simulink model "SimulinkAnalysisofCheetahTail"  (R2022a)
settings: Solver=ode4  StartTime=0.0  StopTime=1.5  FixedStep=0.001  RelTol=1e-3
undefined symbols (not defined in the file): B_cg_H, B_con_H, B_con_L, bar_len, cd_table, Cf, cl_table, g, gear_ratio, int_point_bar, int_point_tail, ITail, M_add, M_cg_H, M_cg_L, M_cg_W, Mb, Mm, Mt, psi3, rho, T_cg_H, T_fur_gap, T_length, T_width_major, T_width_minor, th2_initial, torque_constant, uncertainty_Forces, uncertainty_Position, Vf, windspeed
(part 11 of 21)

== matlab function SimulinkAnalysisofCheetahTail/Model/GravityMatrix ==
  data: B_cg_H parameter; B_con_H parameter; B_con_L parameter; M_cg_H parameter; M_cg_L parameter; M_cg_W parameter; Mb parameter; Mm parameter; Mt parameter; T_cg_H parameter; g parameter; G output; q input
function G = GravityMatrix(B_cg_H,B_con_H,B_con_L,M_cg_H,M_cg_L,M_cg_W,Mb,Mm,Mt,T_cg_H,g,q)
%#codegen
[x,y,z,phi1,th1,psi1,phi2,th2] = deal(q(1),q(2),q(3),q(4),q(5),q(6),q(7),q(8));
% [dx,dy,dz,dphi1,dth1,dpsi1,dphi2,dth2] = deal(dq(1),dq(2),dq(3),dq(4),dq(5),dq(6),dq(7),dq(8));
%    This function was generated by the Symbolic Math Toolbox version 9.0.
%    26-Jan-2022 10:48:01

t2 = cos(phi1);
t3 = cos(phi2);
t4 = cos(th1);
t5 = cos(th2);
t6 = sin(phi1);
t7 = sin(phi2);
t8 = sin(th1);
t9 = sin(th2);
t10 = M_cg_L+x;
t11 = M_cg_W+y;
t12 = M_cg_H+z;
t13 = B_con_L.*t4;
t14 = t4.*t10;
t15 = B_con_H.*t2.*t8;
t16 = B_con_H.*t4.*t6;
t17 = t6.*t7.*t8;
t18 = t7.*t8.*t9;
t19 = t2.*t4.*t7;
t20 = t3.*t4.*t6;
t21 = t3.*t4.*t9;
t22 = t3.*t5.*t8;
t23 = t2.*t4.*t11;
t24 = t2.*t8.*t12;
t25 = t4.*t6.*t12;
t26 = t6.*t8.*t11;
t27 = -t15;
t28 = -t17;
t29 = -t18;
t30 = t2.*t21;
t31 = t2.*t22;
t32 = t5.*t19;
t33 = t5.*t20;
t34 = -t24;
t35 = t19+t33;
t36 = t22+t30;
t37 = t21+t28+t31;
t38 = t20+t29+t32;
mt1 = [Mb.*g.*t8+Mm.*g.*t8+Mt.*g.*t8;-Mb.*g.*t4.*t6-Mm.*g.*t4.*t6-Mt.*g.*t4.*t6;Mb.*g.*t2.*t4+Mm.*g.*t2.*t4+Mt.*g.*t2.*t4;-Mm.*g.*(t23+t25)-Mt.*g.*(t16-t19.*(2.7e+1./1.0e+2)+t23+t25-t33.*(2.7e+1./1.0e+2)-T_cg_H.*t35)-Mb.*g.*(t16+t23+t25-B_cg_H.*t35);Mt.*g.*(t13+t14-t17.*(2.7e+1./1.0e+2)+t21.*(2.7e+1./1.0e+2)+t26+t27+t31.*(2.7e+1./1.0e+2)+t34+T_cg_H.*t37)+Mb.*g.*(t13+t14+t26+t27+t34+B_cg_H.*t37)+Mm.*g.*(t14+t26+t34);0.0];
mt2 = [Mt.*g.*(t18.*(-2.7e+1./1.0e+2)+t20.*(2.7e+1./1.0e+2)+t32.*(2.7e+1./1.0e+2)+T_cg_H.*t38)+B_cg_H.*Mb.*g.*t38;Mt.*g.*(t22.*(2.7e+1./1.0e+2)+t30.*(2.7e+1./1.0e+2)+T_cg_H.*t36)+B_cg_H.*Mb.*g.*t36];
G = [mt1;mt2];

== matlab function SimulinkAnalysisofCheetahTail/Model/ConstraintJacobian ==
  data: A output
function A = ConstraintJacobian
%#codegen

%    This function was generated by the Symbolic Math Toolbox version 9.0.
%    26-Jan-2022 10:48:03

A = reshape([1.0,0.0,0.0,0.0,0.0,0.0,0.0,0.0,1.0,0.0,0.0,0.0,0.0,0.0,0.0,0.0,1.0,0.0,0.0,0.0,0.0,0.0,0.0,0.0,1.0,0.0,0.0,0.0,0.0,0.0,0.0,0.0,1.0,0.0,0.0,0.0,0.0,0.0,0.0,0.0,1.0,0.0,0.0,0.0,0.0,0.0,0.0,0.0,0.0,0.0,0.0,0.0,0.0,0.0,0.0,1.0],[7,8]);

== matlab function SimulinkAnalysisofCheetahTail/Model/ConstraintJacobianDeriv ==
  data: dA output
function dA = ConstraintJacobianDeriv
%#codegen

%    This function was generated by the Symbolic Math Toolbox version 9.0.
%    26-Jan-2022 10:48:04

dA = reshape([0.0,0.0,0.0,0.0,0.0,0.0,0.0,0.0,0.0,0.0,0.0,0.0,0.0,0.0,0.0,0.0,0.0,0.0,0.0,0.0,0.0,0.0,0.0,0.0,0.0,0.0,0.0,0.0,0.0,0.0,0.0,0.0,0.0,0.0,0.0,0.0,0.0,0.0,0.0,0.0,0.0,0.0,0.0,0.0,0.0,0.0,0.0,0.0,0.0,0.0,0.0,0.0,0.0,0.0,0.0,0.0],[7,8]);

== matlab function SimulinkAnalysisofCheetahTail/Model/CalculateLambda ==
  data: M input; lambda output; C input; G input; A input; dA input; Q input; tor input; dq input
function lambda= calcLambda(M,C,G,A,dA,Q, tor, dq)

B = [0;0;0;0;0;0;1;0];
% lambda = -(A*inv(M)*A')\(A*inv(M)*(-C*dq-G)+ dA*dq);
lambda = -((A/M)*A')\((A/M)*(B*tor-C-G-Q)+ dA*dq);

== matlab function SimulinkAnalysisofCheetahTail/Model/Dynamics ==
  data: M input; ddq output; C input; G input; A input; Q input; tor input; lambda input
function ddq = dynamics(M,C,G,A,Q, tor, lambda)
B = [0;0;0;0;0;0;1;0];
% ddq = M\(A'*lambda-C*dq-G);
ddq = M\(A'*lambda+B*tor-C-G-Q);

== matlab function SimulinkAnalysisofCheetahTail/Model/Forces/MATLAB Function ==
  data: int_point_bar input; A_output output; bar_len parameter
function A_output = fcn(int_point_bar, bar_len)

A_output = (bar_len-int_point_bar)*0.02;

== matlab function SimulinkAnalysisofCheetahTail/Model/Forces/NonConstraintForceMatrix_fr ==
  data: Cf parameter; Vf parameter; Q_fr output; q input; dq input
function Q_fr = NonConstraintForceMatrix_fr(Cf,Vf,q, dq)
%#codegen
[x,y,z,phi1,th1,psi1,phi2,th2] = deal(q(1),q(2),q(3),q(4),q(5),q(6),q(7),q(8));
[dx,dy,dz,dphi1,dth1,dpsi1,dphi2,dth2] = deal(dq(1),dq(2),dq(3),dq(4),dq(5),dq(6),dq(7),dq(8));
%    This function was generated by the Symbolic Math Toolbox version 9.0.
%    10-Feb-2022 10:56:36

t2 = cos(psi1);
t3 = cos(th1);
t4 = sin(psi1);
t5 = sin(th1);
t6 = Vf.*dphi2;
t10 = dphi2.*1.0e+1;
t7 = t2.^2;
t8 = t3.^2;
t9 = t4.^2;
t11 = tanh(t10);
t12 = Cf.*t11;
t13 = t6+t12;
Q_fr = [0.0;0.0;0.0;0.0;phi2.*t3.*t5.*t13-phi2.*t3.*t5.*t7.*t13-phi2.*t3.*t5.*t9.*t13;0.0;t5.^2.*t13+t7.*t8.*t13+t8.*t9.*t13;0.0];

== matlab function SimulinkAnalysisofCheetahTail/Model/Forces/NonConstraintForceMatrix_bar ==
  data: B_con_H parameter; B_con_L parameter; M_cg_H parameter; M_cg_L parameter; M_cg_W parameter; area_bar_drag input; bar_len parameter; int_point_bar input; psi3 parameter; rho parameter; windspeed parameter; q input; dq input; Q_bar output
function Q_bar = NonConstraintForceMatrix_bar(B_con_H,B_con_L,M_cg_H,M_cg_L,M_cg_W,area_bar_drag,bar_len,int_point_bar,psi3,rho,windspeed,q,dq)
%#codegen
[x,y,z,phi1,th1,psi1,phi2,th2] = deal(q(1),q(2),q(3),q(4),q(5),q(6),q(7),q(8));
[dx,dy,dz,dphi1,dth1,dpsi1,dphi2,dth2] = deal(dq(1),dq(2),dq(3),dq(4),dq(5),dq(6),dq(7),dq(8));
%    This function was generated by the Symbolic Math Toolbox version 9.0.
%    09-Feb-2022 08:48:45

t2 = cos(phi1);
t3 = cos(phi2);
t4 = cos(psi1);
t5 = cos(psi3);
t6 = cos(th1);
t7 = cos(th2);
t8 = sin(phi1);
t9 = sin(phi2);
t10 = sin(psi1);
t11 = sin(psi3);
t12 = sin(th1);
t13 = sin(th2);
t14 = M_cg_L+x;
t15 = M_cg_W+y;
t16 = M_cg_H+z;
t26 = bar_len./2.0;
t27 = int_point_bar./2.0;
t17 = B_con_L.*t6;
t18 = B_con_L.*t12;
t19 = t2.*t4;
t20 = t6.*t7;
t21 = t2.*t10;
t22 = t4.*t8;
t23 = t7.*t12;
t24 = t8.*t10;
t25 = t12.*t13;
t28 = B_con_H.*t2.*t6;
t30 = t6.*t14;
t31 = B_con_H.*t2.*t12;
t32 = B_con_H.*t6.*t8;
t35 = t12.*t14;
t39 = t6.*t9.*t13;
t41 = t6.*t10.*t13;
t43 = t8.*t9.*t12;
t46 = t2.*t3.*t6;
t49 = t2.*t6.*t9;
t50 = t3.*t6.*t8;
t52 = t2.*t6.*t13;
t53 = t3.*t6.*t13;
t55 = t4.*t6.*t13;
t58 = t3.*t8.*t12;
t59 = t6.*t8.*t9;
t64 = t2.*t6.*t15;
t66 = t2.*t6.*t16;
t69 = t6.*t8.*t15;
t70 = t2.*t12.*t16;
t71 = t6.*t8.*t16;
t73 = t8.*t12.*t15;
t127 = t26+t27;
t29 = t4.*t17;
t33 = t4.*t18;
t34 = t10.*t17;
t36 = t10.*t18;
t37 = t2.*t25;
t38 = t3.*t25;
t40 = t9.*t23;
t42 = t10.*t23;
t44 = t12.*t24;
t45 = t9.*t25;
t47 = t2.*t20;
t48 = t4.*t20;
t51 = t12.*t19;
t54 = t3.*t23;
t56 = t4.*t23;
t57 = t10.*t20;
t60 = t12.*t21;
t61 = t12.*t22;
t62 = B_con_H.*t6.*t19;
t63 = t4.*t30;
t65 = B_con_H.*t6.*t21;
t67 = t4.*t35;
t68 = t10.*t30;
t72 = t10.*t35;
t74 = -t31;
t77 = -t43;
t82 = t3.*t6.*t22;
t83 = t13.*t46;
t86 = t3.*t8.*t20;
t87 = t6.*t13.*t19;
t88 = t4.*t53;
t91 = t3.*t6.*t24;
t92 = t6.*t9.*t22;
t93 = t2.*t39;
t95 = t8.*t9.*t20;
t96 = t6.*t13.*t21;
t98 = t3.*t41;
t99 = t4.*t39;
t101 = t6.*t9.*t24;
t105 = t10.*t39;
t107 = -t55;
t110 = t6.*t16.*t19;
t111 = t6.*t15.*t22;
t112 = t6.*t16.*t21;
t113 = t6.*t15.*t24;
t115 = -t69;
t116 = -t70;
t117 = t3.*t19.*t20;
t118 = t3.*t20.*t21;
t119 = t9.*t19.*t20;
t120 = t9.*t20.*t21;
t131 = t23+t52;
t75 = -t34;
t76 = -t37;
t78 = -t44;
t79 = -t45;
t80 = t3.*t47;
t81 = t3.*t48;
t84 = t2.*t54;
t85 = t9.*t47;
t89 = t3.*t57;
t90 = t9.*t48;
t94 = t2.*t40;
t97 = t4.*t38;
t100 = t9.*t57;
t102 = -t47;
t103 = t10.*t38;
t104 = t4.*t45;
t106 = -t51;
t108 = -t57;
t109 = t10.*t45;
t114 = -t68;
t122 = -t88;
t124 = -t95;
t129 = -t111;
t130 = -t113;
t132 = t21+t61;
t133 = t22+t60;
t134 = -t117;
t135 = -t118;
t145 = t12.*t131;
t149 = t49+t86;
t152 = t54+t83;
t153 = t56+t87;
t154 = t40+t93;
t155 = t42+t96;
t160 = t2.*t6.*t131;
t163 = t6.*t8.*t131;
t121 = -t80;
t123 = -t89;
t125 = -t100;
t126 = t4.*t79;
t128 = t10.*t79;
t136 = B_con_H.*t132;
t137 = B_con_H.*t133;
t138 = t20+t76;
t139 = t25+t102;
t140 = t19+t78;
t141 = t24+t106;
t142 = t3.*t132;
t143 = t3.*t133;
t144 = t7.*t133;
t146 = t9.*t132;
t147 = t9.*t133;
t148 = t13.*t133;
t156 = t15.*t132;
t157 = t15.*t133;
t158 = t16.*t132;
t159 = t16.*t133;
t174 = t46+t124;
t183 = -t163;
t193 = t39+t58+t94;
t196 = t53+t77+t84;
t197 = t50+t79+t85;
t201 = t127.*t149;
t218 = t92+t97+t134;
t221 = t101+t103+t135;
t234 = t127.*t131.*t152;
t150 = B_con_H.*t140;
t151 = B_con_H.*t141;
t161 = t7.*t142;
t162 = t7.*t143;
t164 = t13.*t143;
t165 = t7.*t146;
t166 = t9.*t144;
t167 = t13.*t147;
t168 = t3.*t140;
t169 = t3.*t141;
t170 = t7.*t141;
t171 = t9.*t140;
t172 = t9.*t141;
t173 = t13.*t141;
t175 = t15.*t140;
t176 = t15.*t141;
t177 = -t157;
t178 = t16.*t140;
t179 = t16.*t141;
t192 = t41+t144;
t194 = t108+t148;
t195 = t38+t59+t121;
t199 = t197.^2;
t203 = t12.*t197;
t206 = -t5.*windspeed.*(t57-t148);
t212 = -t6.*t10.*(t57-t148);
t213 = t2.*t6.*t197;
t215 = t6.*t8.*t197;
t216 = -t201;
t219 = t82+t119+t126;
t222 = t91+t120+t128;
t224 = t6.*t10.*(t57-t148);
t228 = t127.*t196;
t233 = -t133.*(t57-t148);
t236 = -t140.*(t57-t148);
t237 = t127.*t221;
t238 = t127.*t218;
t249 = t127.*t131.*t197;
t260 = t127.*t152.*t197;
t180 = t7.*t168;
t181 = t7.*t169;
t182 = -t161;
t184 = t13.*t169;
t185 = t7.*t171;
t186 = t9.*t170;
t187 = t13.*t172;
t188 = -t168;
t189 = -t176;
t198 = t48+t173;
t200 = t107+t170;
t202 = t12.*t195;
t205 = t123+t164;
t209 = t125+t167;
t211 = t2.*t6.*t195;
t214 = t6.*t8.*t195;
t217 = -t203;
t226 = t165+t169;
t227 = t127.*t195;
t231 = t127.*t199;
t239 = t98+t162+t171;
t248 = -t127.*(t161-t172);
t257 = t32+t64+t71+t216;
t261 = -t260;
t279 = t127.*(t57-t148).*(t89-t164);
t284 = t17+t30+t73+t74+t116+t228;
t296 = t33+t62+t67+t110+t129+t238;
t300 = t36+t65+t72+t112+t130+t237;
t190 = -t180;
t191 = -t186;
t204 = t81+t184;
t207 = t11.*t198.*windspeed;
t208 = t90+t187;
t210 = t4.*t6.*t198;
t223 = -t211;
t225 = t143+t185;
t230 = t172+t182;
t232 = t132.*t198;
t235 = t141.*t198;
t240 = t122+t146+t181;
t242 = t105+t166+t188;
t243 = t5.*t239.*windspeed;
t246 = t6.*t10.*t239;
t259 = t152.*t227;
t262 = t127.*t239;
t263 = t133.*t239;
t270 = t140.*t239;
t276 = t197.*t227;
t280 = t131.*t257;
t283 = t18+t28+t35+t66+t115+t227;
t286 = t195.*t257;
t287 = t197.*t257;
t299 = t131.*t284;
t319 = t195.*t284;
t320 = t197.*t284;
t324 = t136+t158+t189+t248;
t330 = -t300.*(t57-t148);
t331 = t198.*t296;
t337 = t239.*t300;
t220 = -t207;
t229 = t147+t190;
t241 = t99+t142+t191;
t245 = t242.^2;
t250 = t11.*t240.*windspeed;
t251 = -t243;
t252 = t5.*t242.*windspeed;
t254 = t4.*t6.*t240;
t256 = t6.*t10.*t242;
t264 = t127.*t240;
t265 = -t262;
t268 = t132.*t240;
t271 = t133.*t242;
t273 = t141.*t240;
t275 = t140.*t242;
t281 = t127.*t198.*t204;
t282 = -t280;
t285 = t6.*t8.*t13.*t283;
t288 = t145+t210+t224;
t291 = -t287;
t293 = -t127.*t242.*(t57-t148);
t297 = t138.*t283;
t298 = t139.*t283;
t303 = t262.*(t89-t164);
t304 = -t127.*t242.*(t89-t164);
t305 = t154.*t283;
t307 = t149.*t283;
t308 = t152.*t283;
t310 = t127.*t242.*(t89-t164);
t311 = t174.*t283;
t313 = t193.*t283;
t315 = t195.*t283;
t316 = t196.*t283;
t317 = t197.*t283;
t318 = t160+t233+t235;
t323 = t183+t232+t236;
t325 = -dy.*(t163-t232+t140.*(t57-t148));
t326 = t242.*t262;
t332 = -t331;
t335 = t198.*t324;
t339 = -t337;
t340 = t242.*t300;
t342 = t240.*t296;
t349 = -t155.*(t34+t68-t137-t159-t175+t262);
t350 = -t13.*t140.*(t34+t68-t137-t159-t175+t262);
t352 = t240.*t324;
t355 = -t192.*(t34+t68-t137-t159-t175+t262);
t368 = (t89-t164).*(t34+t68-t137-t159-t175+t262);
t369 = (t100-t167).*(t34+t68-t137-t159-t175+t262);
t375 = -t221.*(t34+t68-t137-t159-t175+t262);
t376 = -t222.*(t34+t68-t137-t159-t175+t262);
t381 = -t225.*(t34+t68-t137-t159-t175+t262);
t386 = -t239.*(t34+t68-t137-t159-t175+t262);
t389 = -t242.*(t34+t68-t137-t159-t175+t262);
t244 = t241.^2;
t247 = t127.*t229;
t253 = t11.*t241.*windspeed;
t255 = t4.*t6.*t241;
t258 = -t254;
t267 = t127.*t245;
t269 = t132.*t241;
t272 = -t264;
t274 = t141.*t241;
t278 = -t275;
t289 = -t285;
t290 = dx.*t288;
t292 = t127.*t198.*t241;
t294 = t265.*(t89-t164);
t301 = t204.*t264;
t302 = t127.*t204.*t241;
t306 = -t298;
t312 = -t307;
t314 = -t313;
t321 = -t315;
t322 = dz.*t318;
t328 = t241.*t264;
t329 = t242.*t265;
t334 = t75+t114+t137+t159+t175+t265;
t344 = t241.*t296;
t354 = t241.*t324;
t356 = t214+t268+t270;
t360 = t223+t263+t273;
t383 = -t229.*(t34+t68-t137-t159-t175+t262);
t385 = t229.*(t34+t68-t137-t159-t175+t262);
t266 = t127.*t244;
t277 = -t274;
t295 = -t292;
t309 = t204.*t272;
t327 = t150+t177+t178+t247;
t333 = t29+t63+t151+t156+t179+t272;
t338 = t202+t246+t258;
t343 = t217+t255+t256;
t357 = -t354;
t359 = dy.*t356;
t363 = t215+t269+t278;
t364 = dz.*t360;
t392 = -dphi2.*(-t249+t292+t127.*t242.*(t57-t148));
t336 = -t327.*(t57-t148);
t341 = dx.*t338;
t345 = dx.*t343;
t347 = t13.*t132.*t333;
t348 = t153.*t333;
t353 = t239.*t327;
t358 = t242.*t327;
t361 = -t333.*(t55-t170);
t362 = t213+t271+t277;
t365 = -t359;
t366 = t204.*t333;
t367 = t208.*t333;
t370 = -t364;
t372 = dy.*t363;
t373 = t218.*t333;
t374 = t219.*t333;
t380 = t226.*t333;
t382 = -t333.*(t161-t172);
t384 = t333.*(t161-t172);
t387 = t240.*t333;
t388 = t241.*t333;
t391 = t249+t293+t295;
t346 = -t345;
t351 = -t348;
t371 = dz.*t362;
t377 = -t372;
t378 = -t373;
t379 = -t374;
t390 = -t388;
t393 = t234+t279+t281+t306+t355+t361;
t395 = t231+t266+t267+t321+t386+t387;
t397 = t259+t303+t308+t309+t366+t368;
t398 = t261+t302+t305+t310+t367+t369;
t403 = t282+t289+t335+t336+t347+t350;
t404 = -dth1.*(-t297-t299+t331+t348+t155.*(t34+t68-t137-t159-t175+t262)+t300.*(t57-t148));
t405 = -dphi1.*(t280+t285-t335-t347+t327.*(t57-t148)+t13.*t140.*(t34+t68-t137-t159-t175+t262));
t407 = -dphi2.*(-t276-t317+t326+t388+t242.*(t34+t68-t137-t159-t175+t262)+t241.*t272);
t410 = -dth1.*(t313-t320-t340-t344+t374+t222.*(t34+t68-t137-t159-t175+t262));
t412 = t291+t311+t357+t358+t380+t381;
t413 = -dphi1.*(t287-t311+t354-t358-t380+t225.*(t34+t68-t137-t159-t175+t262));
t414 = t286+t312+t352+t353+t384+t385;
t394 = dth2.*t393;
t396 = dphi2.*t395;
t399 = dth2.*t397;
t400 = dth2.*t398;
t402 = t297+t299+t330+t332+t349+t351;
t406 = t276+t317+t328+t329+t389+t390;
t408 = t316+t319+t339+t342+t375+t378;
t409 = t314+t320+t340+t344+t376+t379;
t415 = dphi1.*t414;
t401 = -t400;
t411 = dth1.*t408;
t416 = -t415;
t417 = t206+t220+t290+t322+t325+t392+t394+t404+t405;
t423 = -1.0./(-t252-t253+t345-t371+t372-t396+t400+dphi1.*(t287-t311+t354-t358-t380+t225.*(t34+t68-t137-t159-t175+t262))+dth1.*(t313-t320-t340-t344+t374+t222.*(t34+t68-t137-t159-t175+t262)));
t418 = abs(t417);
t420 = t252+t253+t346+t371+t377+t396+t401+t410+t413;
t424 = t250+t251+t341+t365+t370+t399+t407+t411+t416;
t427 = (t243-t250-t341+t359+t364-t399-t411+t415+dphi2.*(-t276-t317+t326+t388+t242.*(t34+t68-t137-t159-t175+t262)+t241.*t272))./(-t252-t253+t345-t371+t372-t396+t400+dphi1.*(t287-t311+t354-t358-t380+t225.*(t34+t68-t137-t159-t175+t262))+dth1.*(t313-t320-t340-t344+t374+t222.*(t34+t68-t137-t159-t175+t262)));
t419 = t418.^2;
t421 = abs(t420);
t425 = abs(t424);
t428 = atan(t427);
t422 = t421.^2;
t426 = t425.^2;
t429 = -t428;
t430 = t429+th2;
t432 = t419+t422+t426;
t431 = cos(t430);
t433 = sqrt(t432);
t434 = area_bar_drag.*rho.*t131.*t431.*t433.*(t207-t290-t322-t394+dth1.*(-t297-t299+t331+t348+t155.*(t34+t68-t137-t159-t175+t262)+t300.*(t57-t148))+dphi2.*(-t249+t292+t127.*t242.*(t57-t148))+dphi1.*(t280+t285-t335-t347+t327.*(t57-t148)+t13.*t140.*(t34+t68-t137-t159-t175+t262))+dy.*(t163-t232+t140.*(t57-t148))+t5.*windspeed.*(t57-t148)).*(-2.1e+1./2.0e+1);
t435 = rho.*t131.*t431.*t433.*(t207-t290-t322-t394+dth1.*(-t297-t299+t331+t348+t155.*(t34+t68-t137-t159-t175+t262)+t300.*(t57-t148))+dphi2.*(-t249+t292+t127.*t242.*(t57-t148))+dphi1.*(t280+t285-t335-t347+t327.*(t57-t148)+t13.*t140.*(t34+t68-t137-t159-t175+t262))+dy.*(t163-t232+t140.*(t57-t148))+t5.*windspeed.*(t57-t148)).*(-4.2e-4);
t436 = area_bar_drag.*rho.*t198.*t431.*t433.*(t207-t290-t322-t394+dth1.*(-t297-t299+t331+t348+t155.*(t34+t68-t137-t159-t175+t262)+t300.*(t57-t148))+dphi2.*(-t249+t292+t127.*t242.*(t57-t148))+dphi1.*(t280+t285-t335-t347+t327.*(t57-t148)+t13.*t140.*(t34+t68-t137-t159-t175+t262))+dy.*(t163-t232+t140.*(t57-t148))+t5.*windspeed.*(t57-t148)).*(-2.1e+1./2.0e+1);
t437 = area_bar_drag.*rho.*t431.*t433.*(t57-t148).*(t207-t290-t322-t394+dth1.*(-t297-t299+t331+t348+t155.*(t34+t68-t137-t159-t175+t262)+t300.*(t57-t148))+dphi2.*(-t249+t292+t127.*t242.*(t57-t148))+dphi1.*(t280+t285-t335-t347+t327.*(t57-t148)+t13.*t140.*(t34+t68-t137-t159-t175+t262))+dy.*(t163-t232+t140.*(t57-t148))+t5.*windspeed.*(t57-t148)).*(2.1e+1./2.0e+1);
t438 = area_bar_drag.*rho.*t198.*t431.*t433.*(t207-t290-t322-t394+dth1.*(-t297-t299+t331+t348+t155.*(t34+t68-t137-t159-t175+t262)+t300.*(t57-t148))+dphi2.*(-t249+t292+t127.*t242.*(t57-t148))+dphi1.*(t280+t285-t335-t347+t327.*(t57-t148)+t13.*t140.*(t34+t68-t137-t159-t175+t262))+dy.*(t163-t232+t140.*(t57-t148))+t5.*windspeed.*(t57-t148)).*(2.1e+1./2.0e+1);
t439 = rho.*t198.*t431.*t433.*(t207-t290-t322-t394+dth1.*(-t297-t299+t331+t348+t155.*(t34+t68-t137-t159-t175+t262)+t300.*(t57-t148))+dphi2.*(-t249+t292+t127.*t242.*(t57-t148))+dphi1.*(t280+t285-t335-t347+t327.*(t57-t148)+t13.*t140.*(t34+t68-t137-t159-t175+t262))+dy.*(t163-t232+t140.*(t57-t148))+t5.*windspeed.*(t57-t148)).*(-4.2e-4);
t440 = rho.*t431.*t433.*(t57-t148).*(t207-t290-t322-t394+dth1.*(-t297-t299+t331+t348+t155.*(t34+t68-t137-t159-t175+t262)+t300.*(t57-t148))+dphi2.*(-t249+t292+t127.*t242.*(t57-t148))+dphi1.*(t280+t285-t335-t347+t327.*(t57-t148)+t13.*t140.*(t34+t68-t137-t159-t175+t262))+dy.*(t163-t232+t140.*(t57-t148))+t5.*windspeed.*(t57-t148)).*4.2e-4;
t441 = rho.*t198.*t431.*t433.*(t207-t290-t322-t394+dth1.*(-t297-t299+t331+t348+t155.*(t34+t68-t137-t159-t175+t262)+t300.*(t57-t148))+dphi2.*(-t249+t292+t127.*t242.*(t57-t148))+dphi1.*(t280+t285-t335-t347+t327.*(t57-t148)+t13.*t140.*(t34+t68-t137-t159-t175+t262))+dy.*(t163-t232+t140.*(t57-t148))+t5.*windspeed.*(t57-t148)).*4.2e-4;
t442 = rho.*t431.*t433.*(-t252-t253+t345-t371+t372-t396+t400+dphi1.*(t287-t311+t354-t358-t380+t225.*(t34+t68-t137-t159-t175+t262))+dth1.*(t313-t320-t340-t344+t374+t222.*(t34+t68-t137-t159-t175+t262))).*(-4.2e-4);
t443 = area_bar_drag.*rho.*t197.*t431.*t433.*(-t252-t253+t345-t371+t372-t396+t400+dphi1.*(t287-t311+t354-t358-t380+t225.*(t34+t68-t137-t159-t175+t262))+dth1.*(t313-t320-t340-t344+t374+t222.*(t34+t68-t137-t159-t175+t262))).*(-2.1e+1./2.0e+1);
t444 = area_bar_drag.*rho.*t241.*t431.*t433.*(-t252-t253+t345-t371+t372-t396+t400+dphi1.*(t287-t311+t354-t358-t380+t225.*(t34+t68-t137-t159-t175+t262))+dth1.*(t313-t320-t340-t344+t374+t222.*(t34+t68-t137-t159-t175+t262))).*(-2.1e+1./2.0e+1);
t445 = area_bar_drag.*rho.*t242.*t431.*t433.*(-t252-t253+t345-t371+t372-t396+t400+dphi1.*(t287-t311+t354-t358-t380+t225.*(t34+t68-t137-t159-t175+t262))+dth1.*(t313-t320-t340-t344+t374+t222.*(t34+t68-t137-t159-t175+t262))).*(-2.1e+1./2.0e+1);
t446 = rho.*t431.*t433.*(-t252-t253+t345-t371+t372-t396+t400+dphi1.*(t287-t311+t354-t358-t380+t225.*(t34+t68-t137-t159-t175+t262))+dth1.*(t313-t320-t340-t344+t374+t222.*(t34+t68-t137-t159-t175+t262))).*(-2.571758278209442e-20);
t447 = rho.*t431.*t433.*(t243-t250-t341+t359+t364-t399-t411+t415+dphi2.*(-t276-t317+t326+t388+t242.*(t34+t68-t137-t159-t175+t262)+t241.*t272)).*(-4.2e-4);
t448 = rho.*t431.*t433.*(t243-t250-t341+t359+t364-t399-t411+t415+dphi2.*(-t276-t317+t326+t388+t242.*(t34+t68-t137-t159-t175+t262)+t241.*t272)).*4.2e-4;
t449 = area_bar_drag.*rho.*t195.*t431.*t433.*(t243-t250-t341+t359+t364-t399-t411+t415+dphi2.*(-t276-t317+t326+t388+t242.*(t34+t68-t137-t159-t175+t262)+t241.*t272)).*(-2.1e+1./2.0e+1);
t450 = area_bar_drag.*rho.*t239.*t431.*t433.*(t243-t250-t341+t359+t364-t399-t411+t415+dphi2.*(-t276-t317+t326+t388+t242.*(t34+t68-t137-t159-t175+t262)+t241.*t272)).*(-2.1e+1./2.0e+1);
t451 = area_bar_drag.*rho.*t239.*t431.*t433.*(t243-t250-t341+t359+t364-t399-t411+t415+dphi2.*(-t276-t317+t326+t388+t242.*(t34+t68-t137-t159-t175+t262)+t241.*t272)).*(2.1e+1./2.0e+1);
t452 = area_bar_drag.*rho.*t240.*t431.*t433.*(t243-t250-t341+t359+t364-t399-t411+t415+dphi2.*(-t276-t317+t326+t388+t242.*(t34+t68-t137-t159-t175+t262)+t241.*t272)).*(-2.1e+1./2.0e+1);
t453 = rho.*t431.*t433.*(t243-t250-t341+t359+t364-t399-t411+t415+dphi2.*(-t276-t317+t326+t388+t242.*(t34+t68-t137-t159-t175+t262)+t241.*t272)).*(-2.571758278209442e-20);
et1 = rho.*t431.*t433.*(t243-t250-t341+t359+t364-t399-t411+t415+dphi2.*(-t276-t317+t326+t388+t242.*(t34+t68-t137-t159-t175+t262)+t241.*t272)).*2.571758278209442e-20;
et2 = rho.*t431.*t433.*(-t252-t253+t345-t371+t372-t396+t400+dphi1.*(t287-t311+t354-t358-t380+t225.*(t34+t68-t137-t159-t175+t262))+dth1.*(t313-t320-t340-t344+t374+t222.*(t34+t68-t137-t159-t175+t262))).*4.2e-4;
t456 = -t195.*(et1+et2);
et3 = rho.*t431.*t433.*(t243-t250-t341+t359+t364-t399-t411+t415+dphi2.*(-t276-t317+t326+t388+t242.*(t34+t68-t137-t159-t175+t262)+t241.*t272)).*2.571758278209442e-20;
et4 = rho.*t431.*t433.*(-t252-t253+t345-t371+t372-t396+t400+dphi1.*(t287-t311+t354-t358-t380+t225.*(t34+t68-t137-t159-t175+t262))+dth1.*(t313-t320-t340-t344+t374+t222.*(t34+t68-t137-t159-t175+t262))).*4.2e-4;
t458 = -t239.*(et3+et4);
et5 = rho.*t431.*t433.*(t243-t250-t341+t359+t364-t399-t411+t415+dphi2.*(-t276-t317+t326+t388+t242.*(t34+t68-t137-t159-t175+t262)+t241.*t272)).*2.571758278209442e-20;
et6 = rho.*t431.*t433.*(-t252-t253+t345-t371+t372-t396+t400+dphi1.*(t287-t311+t354-t358-t380+t225.*(t34+t68-t137-t159-t175+t262))+dth1.*(t313-t320-t340-t344+t374+t222.*(t34+t68-t137-t159-t175+t262))).*4.2e-4;
t459 = -t240.*(et5+et6);
et7 = rho.*t431.*t433.*(t243-t250-t341+t359+t364-t399-t411+t415+dphi2.*(-t276-t317+t326+t388+t242.*(t34+t68-t137-t159-t175+t262)+t241.*t272)).*2.571758278209442e-20;
et8 = rho.*t431.*t433.*(-t252-t253+t345-t371+t372-t396+t400+dphi1.*(t287-t311+t354-t358-t380+t225.*(t34+t68-t137-t159-t175+t262))+dth1.*(t313-t320-t340-t344+t374+t222.*(t34+t68-t137-t159-t175+t262))).*4.2e-4;
t460 = t239.*(et7+et8);
t454 = t442+t453;
t455 = t446+t448;
t463 = t434+t443+t449;
t464 = t437+t445+t451;
t465 = t438+t444+t452;
t457 = t197.*t455;
t461 = t241.*t455;
t462 = t242.*t455;
t466 = t435+t456+t457;
t467 = t440+t460+t462;
t468 = t441+t459+t461;
et9 = rho.*t431.*t433.*(t243-t250-t341+t359+t364-t399-t411+t415+dphi2.*(-t276-t317+t326+t388+t242.*(t34+t68-t137-t159-t175+t262)+t241.*t272)).*2.571758278209442e-20;
et10 = rho.*t431.*t433.*(-t252-t253+t345-t371+t372-t396+t400+dphi1.*(t287-t311+t354-t358-t380+t225.*(t34+t68-t137-t159-t175+t262))+dth1.*(t313-t320-t340-t344+t374+t222.*(t34+t68-t137-t159-t175+t262))).*4.2e-4;
et11 = area_bar_drag.*rho.*t195.*t431.*t433.*(t243-t250-t341+t359+t364-t399-t411+t415+dphi2.*(-t276-t317+t326+t388+t242.*(t34+t68-t137-t159-t175+t262)+t241.*t272)).*(2.1e+1./2.0e+1)+area_bar_drag.*rho.*t197.*t431.*t433.*(-t252-t253+t345-t371+t372-t396+t400+dphi1.*(t287-t311+t354-t358-t380+t225.*(t34+t68-t137-t159-t175+t262))+dth1.*(t313-t320-t340-t344+t374+t222.*(t34+t68-t137-t159-t175+t262))).*(2.1e+1./2.0e+1);
et12 = area_bar_drag.*rho.*t131.*t431.*t433.*(t207-t290-t322-t394+dth1.*(-t297-t299+t331+t348+t155.*(t34+t68-t137-t159-t175+t262)+t300.*(t57-t148))+dphi2.*(-t249+t292+t127.*t242.*(t57-t148))+dphi1.*(t280+t285-t335-t347+t327.*(t57-t148)+t13.*t140.*(t34+t68-t137-t159-t175+t262))+dy.*(t163-t232+t140.*(t57-t148))+t5.*windspeed.*(t57-t148)).*(2.1e+1./2.0e+1);
et13 = t12.*(-t457+t195.*(et9+et10)+rho.*t131.*t431.*t433.*(t207-t290-t322-t394+dth1.*(-t297-t299+t331+t348+t155.*(t34+t68-t137-t159-t175+t262)+t300.*(t57-t148))+dphi2.*(-t249+t292+t127.*t242.*(t57-t148))+dphi1.*(t280+t285-t335-t347+t327.*(t57-t148)+t13.*t140.*(t34+t68-t137-t159-t175+t262))+dy.*(t163-t232+t140.*(t57-t148))+t5.*windspeed.*(t57-t148)).*4.2e-4)-t12.*(et11+et12)+t4.*t6.*t468-t6.*t10.*t464+t6.*t10.*t467;
et14 = t4.*t6.*(t436+area_bar_drag.*rho.*t240.*t431.*t433.*(t243-t250-t341+t359+t364-t399-t411+t415+dphi2.*(-t276-t317+t326+t388+t242.*(t34+t68-t137-t159-t175+t262)+t241.*t272)).*(2.1e+1./2.0e+1)+area_bar_drag.*rho.*t241.*t431.*t433.*(-t252-t253+t345-t371+t372-t396+t400+dphi1.*(t287-t311+t354-t358-t380+t225.*(t34+t68-t137-t159-t175+t262))+dth1.*(t313-t320-t340-t344+t374+t222.*(t34+t68-t137-t159-t175+t262))).*(2.1e+1./2.0e+1));
et15 = area_bar_drag.*rho.*t195.*t431.*t433.*(t243-t250-t341+t359+t364-t399-t411+t415+dphi2.*(-t276-t317+t326+t388+t242.*(t34+t68-t137-t159-t175+t262)+t241.*t272)).*(2.1e+1./2.0e+1)+area_bar_drag.*rho.*t197.*t431.*t433.*(-t252-t253+t345-t371+t372-t396+t400+dphi1.*(t287-t311+t354-t358-t380+t225.*(t34+t68-t137-t159-t175+t262))+dth1.*(t313-t320-t340-t344+t374+t222.*(t34+t68-t137-t159-t175+t262))).*(2.1e+1./2.0e+1);
et16 = area_bar_drag.*rho.*t131.*t431.*t433.*(t207-t290-t322-t394+dth1.*(-t297-t299+t331+t348+t155.*(t34+t68-t137-t159-t175+t262)+t300.*(t57-t148))+dphi2.*(-t249+t292+t127.*t242.*(t57-t148))+dphi1.*(t280+t285-t335-t347+t327.*(t57-t148)+t13.*t140.*(t34+t68-t137-t159-t175+t262))+dy.*(t163-t232+t140.*(t57-t148))+t5.*windspeed.*(t57-t148)).*(2.1e+1./2.0e+1);
et17 = rho.*t431.*t433.*(t243-t250-t341+t359+t364-t399-t411+t415+dphi2.*(-t276-t317+t326+t388+t242.*(t34+t68-t137-t159-t175+t262)+t241.*t272)).*2.571758278209442e-20;
et18 = rho.*t431.*t433.*(-t252-t253+t345-t371+t372-t396+t400+dphi1.*(t287-t311+t354-t358-t380+t225.*(t34+t68-t137-t159-t175+t262))+dth1.*(t313-t320-t340-t344+t374+t222.*(t34+t68-t137-t159-t175+t262))).*4.2e-4;
et19 = t132.*t468+t140.*t464-t140.*t467+t132.*(t436+area_bar_drag.*rho.*t240.*t431.*t433.*(t243-t250-t341+t359+t364-t399-t411+t415+dphi2.*(-t276-t317+t326+t388+t242.*(t34+t68-t137-t159-t175+t262)+t241.*t272)).*(2.1e+1./2.0e+1)+area_bar_drag.*rho.*t241.*t431.*t433.*(-t252-t253+t345-t371+t372-t396+t400+dphi1.*(t287-t311+t354-t358-t380+t225.*(t34+t68-t137-t159-t175+t262))+dth1.*(t313-t320-t340-t344+t374+t222.*(t34+t68-t137-t159-t175+t262))).*(2.1e+1./2.0e+1))+t6.*t8.*(et15+et16);
et20 = -t6.*t8.*(-t457+t195.*(et17+et18)+rho.*t131.*t431.*t433.*(t207-t290-t322-t394+dth1.*(-t297-t299+t331+t348+t155.*(t34+t68-t137-t159-t175+t262)+t300.*(t57-t148))+dphi2.*(-t249+t292+t127.*t242.*(t57-t148))+dphi1.*(t280+t285-t335-t347+t327.*(t57-t148)+t13.*t140.*(t34+t68-t137-t159-t175+t262))+dy.*(t163-t232+t140.*(t57-t148))+t5.*windspeed.*(t57-t148)).*4.2e-4);
et21 = area_bar_drag.*rho.*t195.*t431.*t433.*(t243-t250-t341+t359+t364-t399-t411+t415+dphi2.*(-t276-t317+t326+t388+t242.*(t34+t68-t137-t159-t175+t262)+t241.*t272)).*(2.1e+1./2.0e+1)+area_bar_drag.*rho.*t197.*t431.*t433.*(-t252-t253+t345-t371+t372-t396+t400+dphi1.*(t287-t311+t354-t358-t380+t225.*(t34+t68-t137-t159-t175+t262))+dth1.*(t313-t320-t340-t344+t374+t222.*(t34+t68-t137-t159-t175+t262))).*(2.1e+1./2.0e+1);
et22 = area_bar_drag.*rho.*t131.*t431.*t433.*(t207-t290-t322-t394+dth1.*(-t297-t299+t331+t348+t155.*(t34+t68-t137-t159-t175+t262)+t300.*(t57-t148))+dphi2.*(-t249+t292+t127.*t242.*(t57-t148))+dphi1.*(t280+t285-t335-t347+t327.*(t57-t148)+t13.*t140.*(t34+t68-t137-t159-t175+t262))+dy.*(t163-t232+t140.*(t57-t148))+t5.*windspeed.*(t57-t148)).*(2.1e+1./2.0e+1);
et23 = rho.*t431.*t433.*(t243-t250-t341+t359+t364-t399-t411+t415+dphi2.*(-t276-t317+t326+t388+t242.*(t34+t68-t137-t159-t175+t262)+t241.*t272)).*2.571758278209442e-20;
et24 = rho.*t431.*t433.*(-t252-t253+t345-t371+t372-t396+t400+dphi1.*(t287-t311+t354-t358-t380+t225.*(t34+t68-t137-t159-t175+t262))+dth1.*(t313-t320-t340-t344+t374+t222.*(t34+t68-t137-t159-t175+t262))).*4.2e-4;
et25 = t133.*t464-t133.*t467+t141.*t468+t141.*(t436+area_bar_drag.*rho.*t240.*t431.*t433.*(t243-t250-t341+t359+t364-t399-t411+t415+dphi2.*(-t276-t317+t326+t388+t242.*(t34+t68-t137-t159-t175+t262)+t241.*t272)).*(2.1e+1./2.0e+1)+area_bar_drag.*rho.*t241.*t431.*t433.*(-t252-t253+t345-t371+t372-t396+t400+dphi1.*(t287-t311+t354-t358-t380+t225.*(t34+t68-t137-t159-t175+t262))+dth1.*(t313-t320-t340-t344+t374+t222.*(t34+t68-t137-t159-t175+t262))).*(2.1e+1./2.0e+1))-t2.*t6.*(et21+et22);
et26 = t2.*t6.*(-t457+t195.*(et23+et24)+rho.*t131.*t431.*t433.*(t207-t290-t322-t394+dth1.*(-t297-t299+t331+t348+t155.*(t34+t68-t137-t159-t175+t262)+t300.*(t57-t148))+dphi2.*(-t249+t292+t127.*t242.*(t57-t148))+dphi1.*(t280+t285-t335-t347+t327.*(t57-t148)+t13.*t140.*(t34+t68-t137-t159-t175+t262))+dy.*(t163-t232+t140.*(t57-t148))+t5.*windspeed.*(t57-t148)).*4.2e-4);
et27 = rho.*t431.*t433.*(t243-t250-t341+t359+t364-t399-t411+t415+dphi2.*(-t276-t317+t326+t388+t242.*(t34+t68-t137-t159-t175+t262)+t241.*t272)).*2.571758278209442e-20;
et28 = rho.*t431.*t433.*(-t252-t253+t345-t371+t372-t396+t400+dphi1.*(t287-t311+t354-t358-t380+t225.*(t34+t68-t137-t159-t175+t262))+dth1.*(t313-t320-t340-t344+t374+t222.*(t34+t68-t137-t159-t175+t262))).*4.2e-4;
et29 = area_bar_drag.*rho.*t195.*t431.*t433.*(t243-t250-t341+t359+t364-t399-t411+t415+dphi2.*(-t276-t317+t326+t388+t242.*(t34+t68-t137-t159-t175+t262)+t241.*t272)).*(2.1e+1./2.0e+1)+area_bar_drag.*rho.*t197.*t431.*t433.*(-t252-t253+t345-t371+t372-t396+t400+dphi1.*(t287-t311+t354-t358-t380+t225.*(t34+t68-t137-t159-t175+t262))+dth1.*(t313-t320-t340-t344+t374+t222.*(t34+t68-t137-t159-t175+t262))).*(2.1e+1./2.0e+1);
et30 = area_bar_drag.*rho.*t131.*t431.*t433.*(t207-t290-t322-t394+dth1.*(-t297-t299+t331+t348+t155.*(t34+t68-t137-t159-t175+t262)+t300.*(t57-t148))+dphi2.*(-t249+t292+t127.*t242.*(t57-t148))+dphi1.*(t280+t285-t335-t347+t327.*(t57-t148)+t13.*t140.*(t34+t68-t137-t159-t175+t262))+dy.*(t163-t232+t140.*(t57-t148))+t5.*windspeed.*(t57-t148)).*(2.1e+1./2.0e+1);
et31 = -t257.*(-t457+t195.*(et27+et28)+rho.*t131.*t431.*t433.*(t207-t290-t322-t394+dth1.*(-t297-t299+t331+t348+t155.*(t34+t68-t137-t159-t175+t262)+t300.*(t57-t148))+dphi2.*(-t249+t292+t127.*t242.*(t57-t148))+dphi1.*(t280+t285-t335-t347+t327.*(t57-t148)+t13.*t140.*(t34+t68-t137-t159-t175+t262))+dy.*(t163-t232+t140.*(t57-t148))+t5.*windspeed.*(t57-t148)).*4.2e-4)+t327.*t464+t324.*t468-t327.*t467;
et32 = t324.*(t436+area_bar_drag.*rho.*t240.*t431.*t433.*(t243-t250-t341+t359+t364-t399-t411+t415+dphi2.*(-t276-t317+t326+t388+t242.*(t34+t68-t137-t159-t175+t262)+t241.*t272)).*(2.1e+1./2.0e+1)+area_bar_drag.*rho.*t241.*t431.*t433.*(-t252-t253+t345-t371+t372-t396+t400+dphi1.*(t287-t311+t354-t358-t380+t225.*(t34+t68-t137-t159-t175+t262))+dth1.*(t313-t320-t340-t344+t374+t222.*(t34+t68-t137-t159-t175+t262))).*(2.1e+1./2.0e+1))+t257.*(et29+et30);
et33 = rho.*t431.*t433.*(t243-t250-t341+t359+t364-t399-t411+t415+dphi2.*(-t276-t317+t326+t388+t242.*(t34+t68-t137-t159-t175+t262)+t241.*t272)).*2.571758278209442e-20;
Q_bar = ft_1({area_bar_drag,dphi1,dphi2,dth1,dy,et13,et14,et19,et20,et25,et26,et31,et32,et33,rho,t127,t13,t131,t137,t140,t148,t152,t155,t159,t163,t164,t175,t195,t197,t204,t207,t222,t225,t232,t240,t241,t242,t243,t249,t250,t252,t253,t262,t272,t276,t280,t284,t285,t287,t290,t292,t296,t297,t299,t300,t311,t313,t317,t320,t322,t326,t327,t331,t333,t335,t34,t340,t341,t344,t345,t347,t348,t354,t358,t359,t364,t371,t372,t374,t380,t388,t394,t396,t399,t400,t411,t415,t431,t433,t436,t457,t464,t467,t468,t5,t57,t68,t89,windspeed});
end
function Q_bar = ft_1(ct)
area_bar_drag = ct{1};
dphi1 = ct{2};
dphi2 = ct{3};
dth1 = ct{4};
dy = ct{5};
et13 = ct{6};
et14 = ct{7};
et19 = ct{8};
et20 = ct{9};
et25 = ct{10};
et26 = ct{11};
et31 = ct{12};
et32 = ct{13};
et33 = ct{14};
rho = ct{15};
t127 = ct{16};
t13 = ct{17};
t131 = ct{18};
t137 = ct{19};
t140 = ct{20};
t148 = ct{21};
t152 = ct{22};
t155 = ct{23};
t159 = ct{24};
t163 = ct{25};
t164 = ct{26};
t175 = ct{27};
t195 = ct{28};
t197 = ct{29};
t204 = ct{30};
t207 = ct{31};
t222 = ct{32};
t225 = ct{33};
t232 = ct{34};
t240 = ct{35};
t241 = ct{36};
t242 = ct{37};
t243 = ct{38};
t249 = ct{39};
t250 = ct{40};
t252 = ct{41};
t253 = ct{42};
t262 = ct{43};
t272 = ct{44};
t276 = ct{45};
t280 = ct{46};
t284 = ct{47};
t285 = ct{48};
t287 = ct{49};
t290 = ct{50};
t292 = ct{51};
t296 = ct{52};
t297 = ct{53};
t299 = ct{54};
t300 = ct{55};
t311 = ct{56};
t313 = ct{57};
t317 = ct{58};
t320 = ct{59};
t322 = ct{60};
t326 = ct{61};
t327 = ct{62};
t331 = ct{63};
t333 = ct{64};
t335 = ct{65};
t34 = ct{66};
t340 = ct{67};
t341 = ct{68};
t344 = ct{69};
t345 = ct{70};
t347 = ct{71};
t348 = ct{72};
t354 = ct{73};
t358 = ct{74};
t359 = ct{75};
t364 = ct{76};
t371 = ct{77};
t372 = ct{78};
t374 = ct{79};
t380 = ct{80};
t388 = ct{81};
t394 = ct{82};
t396 = ct{83};
t399 = ct{84};
t400 = ct{85};
t411 = ct{86};
t415 = ct{87};
t431 = ct{88};
t433 = ct{89};
t436 = ct{90};
t457 = ct{91};
t464 = ct{92};
t467 = ct{93};
t468 = ct{94};
t5 = ct{95};
t57 = ct{96};
t68 = ct{97};
t89 = ct{98};
windspeed = ct{99};
et34 = rho.*t431.*t433.*(-t252-t253+t345-t371+t372-t396+t400+dphi1.*(t287-t311+t354-t358-t380+t225.*(t34+t68-t137-t159-t175+t262))+dth1.*(t313-t320-t340-t344+t374+t222.*(t34+t68-t137-t159-t175+t262))).*4.2e-4;
et35 = area_bar_drag.*rho.*t195.*t431.*t433.*(t243-t250-t341+t359+t364-t399-t411+t415+dphi2.*(-t276-t317+t326+t388+t242.*(t34+t68-t137-t159-t175+t262)+t241.*t272)).*(2.1e+1./2.0e+1)+area_bar_drag.*rho.*t197.*t431.*t433.*(-t252-t253+t345-t371+t372-t396+t400+dphi1.*(t287-t311+t354-t358-t380+t225.*(t34+t68-t137-t159-t175+t262))+dth1.*(t313-t320-t340-t344+t374+t222.*(t34+t68-t137-t159-t175+t262))).*(2.1e+1./2.0e+1);
et36 = area_bar_drag.*rho.*t131.*t431.*t433.*(t207-t290-t322-t394+dth1.*(-t297-t299+t331+t348+t155.*(t34+t68-t137-t159-t175+t262)+t300.*(t57-t148))+dphi2.*(-t249+t292+t127.*t242.*(t57-t148))+dphi1.*(t280+t285-t335-t347+t327.*(t57-t148)+t13.*t140.*(t34+t68-t137-t159-t175+t262))+dy.*(t163-t232+t140.*(t57-t148))+t5.*windspeed.*(t57-t148)).*(2.1e+1./2.0e+1);
et37 = t284.*(-t457+t195.*(et33+et34)+rho.*t131.*t431.*t433.*(t207-t290-t322-t394+dth1.*(-t297-t299+t331+t348+t155.*(t34+t68-t137-t159-t175+t262)+t300.*(t57-t148))+dphi2.*(-t249+t292+t127.*t242.*(t57-t148))+dphi1.*(t280+t285-t335-t347+t327.*(t57-t148)+t13.*t140.*(t34+t68-t137-t159-t175+t262))+dy.*(t163-t232+t140.*(t57-t148))+t5.*windspeed.*(t57-t148)).*4.2e-4)-t296.*t468+t300.*t464-t300.*t467;
et38 = -t296.*(t436+area_bar_drag.*rho.*t240.*t431.*t433.*(t243-t250-t341+t359+t364-t399-t411+t415+dphi2.*(-t276-t317+t326+t388+t242.*(t34+t68-t137-t159-t175+t262)+t241.*t272)).*(2.1e+1./2.0e+1)+area_bar_drag.*rho.*t241.*t431.*t433.*(-t252-t253+t345-t371+t372-t396+t400+dphi1.*(t287-t311+t354-t358-t380+t225.*(t34+t68-t137-t159-t175+t262))+dth1.*(t313-t320-t340-t344+t374+t222.*(t34+t68-t137-t159-t175+t262))).*(2.1e+1./2.0e+1))-t284.*(et35+et36);
et39 = -t468.*(t34+t68-t137-t159-t175+t262);
et40 = -(t436+area_bar_drag.*rho.*t240.*t431.*t433.*(t243-t250-t341+t359+t364-t399-t411+t415+dphi2.*(-t276-t317+t326+t388+t242.*(t34+t68-t137-t159-t175+t262)+t241.*t272)).*(2.1e+1./2.0e+1)+area_bar_drag.*rho.*t241.*t431.*t433.*(-t252-t253+t345-t371+t372-t396+t400+dphi1.*(t287-t311+t354-t358-t380+t225.*(t34+t68-t137-t159-t175+t262))+dth1.*(t313-t320-t340-t344+t374+t222.*(t34+t68-t137-t159-t175+t262))).*(2.1e+1./2.0e+1)).*(t34+t68-t137-t159-t175+t262)-t333.*t464+t333.*t467;
et41 = area_bar_drag.*rho.*t195.*t431.*t433.*(t243-t250-t341+t359+t364-t399-t411+t415+dphi2.*(-t276-t317+t326+t388+t242.*(t34+t68-t137-t159-t175+t262)+t241.*t272)).*(2.1e+1./2.0e+1)+area_bar_drag.*rho.*t197.*t431.*t433.*(-t252-t253+t345-t371+t372-t396+t400+dphi1.*(t287-t311+t354-t358-t380+t225.*(t34+t68-t137-t159-t175+t262))+dth1.*(t313-t320-t340-t344+t374+t222.*(t34+t68-t137-t159-t175+t262))).*(2.1e+1./2.0e+1);
et42 = area_bar_drag.*rho.*t131.*t431.*t433.*(t207-t290-t322-t394+dth1.*(-t297-t299+t331+t348+t155.*(t34+t68-t137-t159-t175+t262)+t300.*(t57-t148))+dphi2.*(-t249+t292+t127.*t242.*(t57-t148))+dphi1.*(t280+t285-t335-t347+t327.*(t57-t148)+t13.*t140.*(t34+t68-t137-t159-t175+t262))+dy.*(t163-t232+t140.*(t57-t148))+t5.*windspeed.*(t57-t148)).*(2.1e+1./2.0e+1);
et43 = rho.*t431.*t433.*(t243-t250-t341+t359+t364-t399-t411+t415+dphi2.*(-t276-t317+t326+t388+t242.*(t34+t68-t137-t159-t175+t262)+t241.*t272)).*2.571758278209442e-20;
et44 = rho.*t431.*t433.*(-t252-t253+t345-t371+t372-t396+t400+dphi1.*(t287-t311+t354-t358-t380+t225.*(t34+t68-t137-t159-t175+t262))+dth1.*(t313-t320-t340-t344+t374+t222.*(t34+t68-t137-t159-t175+t262))).*4.2e-4;
et45 = -t127.*t197.*(et41+et42)+t127.*t197.*(-t457+t195.*(et43+et44)+rho.*t131.*t431.*t433.*(t207-t290-t322-t394+dth1.*(-t297-t299+t331+t348+t155.*(t34+t68-t137-t159-t175+t262)+t300.*(t57-t148))+dphi2.*(-t249+t292+t127.*t242.*(t57-t148))+dphi1.*(t280+t285-t335-t347+t327.*(t57-t148)+t13.*t140.*(t34+t68-t137-t159-t175+t262))+dy.*(t163-t232+t140.*(t57-t148))+t5.*windspeed.*(t57-t148)).*4.2e-4)+t127.*t242.*t464-t127.*t241.*t468-t127.*t242.*t467;
et46 = -t127.*t241.*(t436+area_bar_drag.*rho.*t240.*t431.*t433.*(t243-t250-t341+t359+t364-t399-t411+t415+dphi2.*(-t276-t317+t326+t388+t242.*(t34+t68-t137-t159-t175+t262)+t241.*t272)).*(2.1e+1./2.0e+1)+area_bar_drag.*rho.*t241.*t431.*t433.*(-t252-t253+t345-t371+t372-t396+t400+dphi1.*(t287-t311+t354-t358-t380+t225.*(t34+t68-t137-t159-t175+t262))+dth1.*(t313-t320-t340-t344+t374+t222.*(t34+t68-t137-t159-t175+t262))).*(2.1e+1./2.0e+1));
et47 = area_bar_drag.*rho.*t195.*t431.*t433.*(t243-t250-t341+t359+t364-t399-t411+t415+dphi2.*(-t276-t317+t326+t388+t242.*(t34+t68-t137-t159-t175+t262)+t241.*t272)).*(2.1e+1./2.0e+1)+area_bar_drag.*rho.*t197.*t431.*t433.*(-t252-t253+t345-t371+t372-t396+t400+dphi1.*(t287-t311+t354-t358-t380+t225.*(t34+t68-t137-t159-t175+t262))+dth1.*(t313-t320-t340-t344+t374+t222.*(t34+t68-t137-t159-t175+t262))).*(2.1e+1./2.0e+1);
et48 = area_bar_drag.*rho.*t131.*t431.*t433.*(t207-t290-t322-t394+dth1.*(-t297-t299+t331+t348+t155.*(t34+t68-t137-t159-t175+t262)+t300.*(t57-t148))+dphi2.*(-t249+t292+t127.*t242.*(t57-t148))+dphi1.*(t280+t285-t335-t347+t327.*(t57-t148)+t13.*t140.*(t34+t68-t137-t159-t175+t262))+dy.*(t163-t232+t140.*(t57-t148))+t5.*windspeed.*(t57-t148)).*(2.1e+1./2.0e+1);
et49 = rho.*t431.*t433.*(t243-t250-t341+t359+t364-t399-t411+t415+dphi2.*(-t276-t317+t326+t388+t242.*(t34+t68-t137-t159-t175+t262)+t241.*t272)).*2.571758278209442e-20;
et50 = rho.*t431.*t433.*(-t252-t253+t345-t371+t372-t396+t400+dphi1.*(t287-t311+t354-t358-t380+t225.*(t34+t68-t137-t159-t175+t262))+dth1.*(t313-t320-t340-t344+t374+t222.*(t34+t68-t137-t159-t175+t262))).*4.2e-4;
et51 = -t127.*t152.*(et47+et48)+t127.*t152.*(-t457+t195.*(et49+et50)+rho.*t131.*t431.*t433.*(t207-t290-t322-t394+dth1.*(-t297-t299+t331+t348+t155.*(t34+t68-t137-t159-t175+t262)+t300.*(t57-t148))+dphi2.*(-t249+t292+t127.*t242.*(t57-t148))+dphi1.*(t280+t285-t335-t347+t327.*(t57-t148)+t13.*t140.*(t34+t68-t137-t159-t175+t262))+dy.*(t163-t232+t140.*(t57-t148))+t5.*windspeed.*(t57-t148)).*4.2e-4)+t127.*t204.*t468;
et52 = t127.*t204.*(t436+area_bar_drag.*rho.*t240.*t431.*t433.*(t243-t250-t341+t359+t364-t399-t411+t415+dphi2.*(-t276-t317+t326+t388+t242.*(t34+t68-t137-t159-t175+t262)+t241.*t272)).*(2.1e+1./2.0e+1)+area_bar_drag.*rho.*t241.*t431.*t433.*(-t252-t253+t345-t371+t372-t396+t400+dphi1.*(t287-t311+t354-t358-t380+t225.*(t34+t68-t137-t159-t175+t262))+dth1.*(t313-t320-t340-t344+t374+t222.*(t34+t68-t137-t159-t175+t262))).*(2.1e+1./2.0e+1))-t127.*t464.*(t89-t164)+t127.*t467.*(t89-t164);
Q_bar = [et13+et14;et19+et20;et25+et26;et31+et32;et37+et38;et39+et40;et45+et46;et51+et52];
end
